simulink model "simulink_model_closed_loop"  (R2019a)
settings: Solver=VariableStepAuto  StartTime=0.0  StopTime=100.0  RelTol=1e-3
values from neighbouring files (symbols this model uses):
  lbu = [dbeta_min; dM_gen_min]    [example_closed_loop.m]    (also in example_ocp.m)
  lbx = [OmegaR_min; beta_min; M_gen_min]    [example_closed_loop.m]    (also in example_ocp.m)
  lh = Pel_min    (= 0)    [example_closed_loop.m]    (also in example_ocp.m)
  ubu = [dbeta_max; dM_gen_max]    [example_closed_loop.m]    (also in example_ocp.m)
  ubx = [OmegaR_max; beta_max; M_gen_max]    [example_closed_loop.m]    (also in example_ocp.m)
  uh = Pel_max    (= 5)    [example_closed_loop.m]    (also in example_ocp.m)
  X0 = [statesFAST(1,[9               10                  19                20])                  uCtrlFAST(1,1)      uCtrlFAST(1,2) uCtrlFAST(1,1)       uCtrlFAST(1,2)]    [compute_setup.m]
settings Model: Creator=gianluca  LastModifiedBy=gianluca

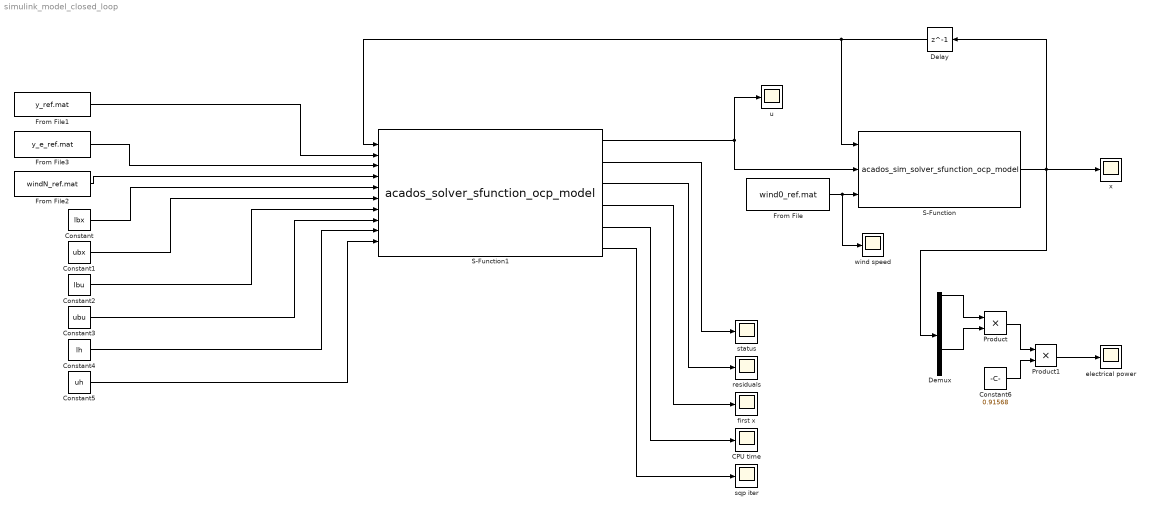
== system simulink_model_closed_loop ==
  CPU time : Scope
  Constant : Constant  Value=lbx
  Constant1 : Constant  Value=ubx
  Constant2 : Constant  Value=lbu
  Constant3 : Constant  Value=ubu
  Constant4 : Constant  Value=lh
  Constant5 : Constant  Value=uh
  Constant6 : Constant  Value=0.91568
  Delay : Delay  DelayLength=1  InitialCondition=X0
  Demux : Demux  Outputs=8
  From File : FromFile  FileName=wind0_ref.mat  SampleTime=0
  From File1 : FromFile  FileName=y_ref.mat  SampleTime=0
  From File2 : FromFile  FileName=windN_ref.mat  SampleTime=0
  From File3 : FromFile  FileName=y_e_ref.mat  SampleTime=0
  Product : Product
  Product1 : Product
  S-Function : S-Function  FunctionName=acados_sim_solver_sfunction_ocp_model  SFunctionDeploymentMode=off  EnableBusSupport=off
  S-Function1 : S-Function  FunctionName=acados_solver_sfunction_ocp_model  SFunctionDeploymentMode=off  EnableBusSupport=off
  electrical power : Scope
  first x : Scope
  residuals : Scope
  "sqp iter " : Scope
  status : Scope
  u : Scope
  wind speed : Scope
  x : Scope
  wires:
  Delay/1 -> S-Function1/1, S-Function/1
  S-Function/1 -> Delay/1, Demux/1, x/1
  Constant3/1 -> S-Function1/8
  Constant2/1 -> S-Function1/7
  Constant1/1 -> S-Function1/6
  Constant/1 -> S-Function1/5
  Constant4/1 -> S-Function1/9
  Constant5/1 -> S-Function1/10
  From File/1 -> wind speed/1, S-Function/3
  From File1/1 -> S-Function1/2
  From File2/1 -> S-Function1/4
  S-Function1/2 -> status/1
  From File3/1 -> S-Function1/3
  Demux/1 -> Product/1
  Demux/6 -> Product/2
  Product/1 -> Product1/1
  Constant6/1 -> Product1/2
  Product1/1 -> electrical power/1
  S-Function1/1 -> S-Function/2, u/1
  S-Function1/6 -> "sqp iter "/1
  S-Function1/5 -> CPU time/1
  S-Function1/4 -> first x/1
  S-Function1/3 -> residuals/1
